simulink library "Lib_AC_AttitudeControl"  (R2014b)
settings: Solver=ode45  StartTime=0.0  StopTime=10.0  RelTol=1e-3
values from neighbouring files (symbols this model uses):
  Cutoff_frequency_roll = 20.0    (= 20)    [LoadParameters.m]    (also in euler_yaw_rate_cd.mat)
  Cutoff_frequency_yaw = 20.0    (= 20)    [LoadParameters.m]
  Discretetime_400Hz = 0.0025    [LoadParameters.m]    (also in euler_yaw_rate_cd.mat)
  roll_rate_kd = 0.0027    [LoadParameters.m]    (also in euler_yaw_rate_cd.mat = 0)
  roll_rate_ki = 0.001    [LoadParameters.m]    (also in euler_yaw_rate_cd.mat = 0)
  roll_rate_kp = 0.12    [LoadParameters.m]    (also in euler_yaw_rate_cd.mat = 0.08)
  yaw_rate_kd = 0.0090    (= 0.009)    [LoadParameters.m]
  yaw_rate_ki = 1.050    (= 1.05)    [LoadParameters.m]
  yaw_rate_kp = 0.45    [LoadParameters.m]
libraries: Lib_AC_PID x3
settings Model: Creator=Ehang  LastModifiedBy=Ehang

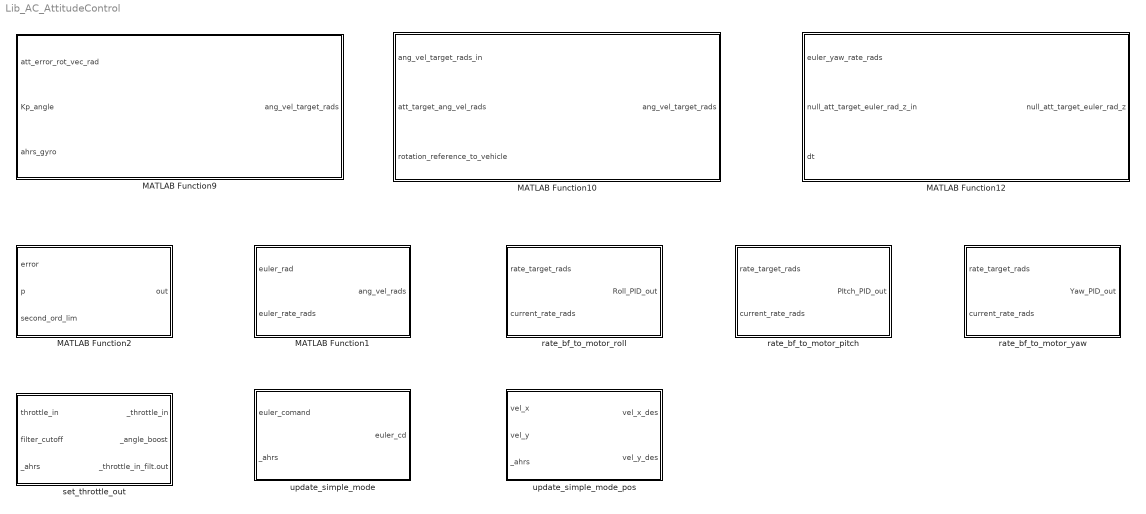
== system Lib_AC_AttitudeControl ==
  MATLAB Function1 : MATLAB Function  TreatAsAtomicUnit=on
  MATLAB Function10 : MATLAB Function  TreatAsAtomicUnit=on
  MATLAB Function12 : MATLAB Function  TreatAsAtomicUnit=on
  MATLAB Function2 : MATLAB Function  TreatAsAtomicUnit=on
  MATLAB Function9 : MATLAB Function  TreatAsAtomicUnit=on
  rate_bf_to_motor_pitch : Subsystem
  rate_bf_to_motor_roll : Subsystem
  rate_bf_to_motor_yaw : Subsystem
  set_throttle_out : Subsystem
  update_simple_mode : Subsystem
  update_simple_mode_pos : Subsystem

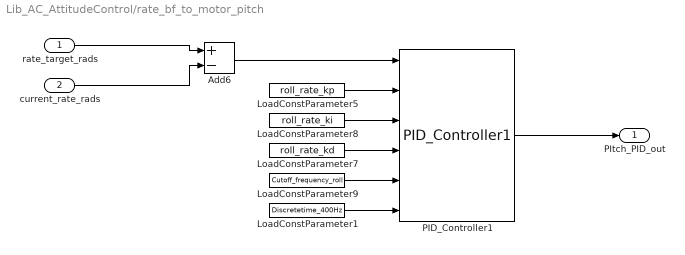
== system Lib_AC_AttitudeControl/rate_bf_to_motor_pitch ==
  rate_target_rads : Inport
  current_rate_rads : Inport  Port=2
  Add6 : Sum  Inputs=+-
  LoadConstParameter1 : Constant  Value=Discretetime_400Hz  SampleTime=-1
  LoadConstParameter5 : Constant  Value=roll_rate_kp  SampleTime=-1
  LoadConstParameter7 : Constant  Value=roll_rate_kd  SampleTime=-1
  LoadConstParameter8 : Constant  Value=roll_rate_ki  SampleTime=-1
  LoadConstParameter9 : Constant  Value=Cutoff_frequency_roll  SampleTime=-1
  PID_Controller1 : Lib_AC_PID/PID_Controller1  Description=PI控制器。
  PItch_PID_out : Outport
  wires:
  PID_Controller1/1 -> PItch_PID_out/1
  LoadConstParameter1/1 -> PID_Controller1/6
  LoadConstParameter9/1 -> PID_Controller1/5
  LoadConstParameter7/1 -> PID_Controller1/4
  LoadConstParameter8/1 -> PID_Controller1/3
  LoadConstParameter5/1 -> PID_Controller1/2
  Add6/1 -> PID_Controller1/1
  current_rate_rads/1 -> Add6/2
  rate_target_rads/1 -> Add6/1

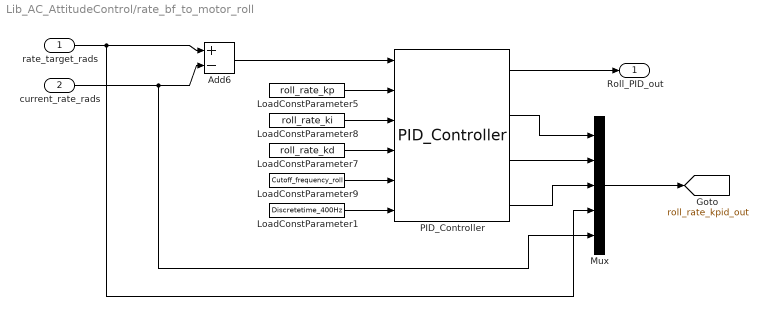
== system Lib_AC_AttitudeControl/rate_bf_to_motor_roll ==
  rate_target_rads : Inport
  current_rate_rads : Inport  Port=2
  Add6 : Sum  Inputs=+-
  LoadConstParameter1 : Constant  Value=Discretetime_400Hz  SampleTime=-1
  LoadConstParameter5 : Constant  Value=roll_rate_kp  SampleTime=-1
  LoadConstParameter7 : Constant  Value=roll_rate_kd  SampleTime=-1
  LoadConstParameter8 : Constant  Value=roll_rate_ki  SampleTime=-1
  LoadConstParameter9 : Constant  Value=Cutoff_frequency_roll  SampleTime=-1
  Mux : Mux  Inputs=5
  PID_Controller : Lib_AC_PID/PID_Controller  Description=PI控制器。
  Roll_PID_out : Outport
  tag scope: roll_rate_kpid_out=global
  wires:
  Mux/1 -> [roll_rate_kpid_out]
  PID_Controller/4 -> Mux/3
  PID_Controller/2 -> Mux/1
  PID_Controller/3 -> Mux/2
  PID_Controller/1 -> Roll_PID_out/1
  LoadConstParameter1/1 -> PID_Controller/6
  LoadConstParameter9/1 -> PID_Controller/5
  LoadConstParameter7/1 -> PID_Controller/4
  LoadConstParameter8/1 -> PID_Controller/3
  LoadConstParameter5/1 -> PID_Controller/2
  Add6/1 -> PID_Controller/1
  current_rate_rads/1 -> Mux/5, Add6/2
  rate_target_rads/1 -> Mux/4, Add6/1

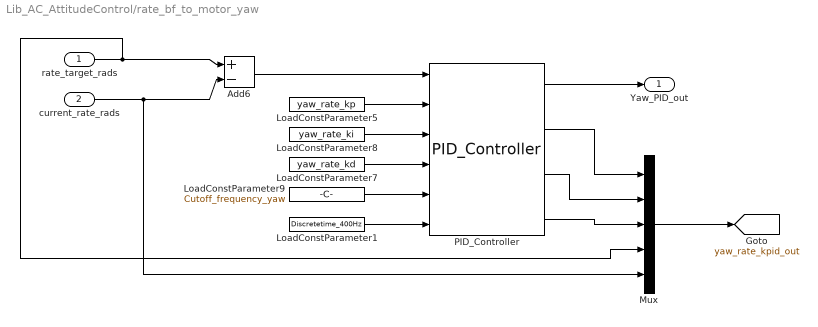
== system Lib_AC_AttitudeControl/rate_bf_to_motor_yaw ==
  rate_target_rads : Inport
  current_rate_rads : Inport  Port=2
  Add6 : Sum  Inputs=+-
  LoadConstParameter1 : Constant  Value=Discretetime_400Hz  SampleTime=-1
  LoadConstParameter5 : Constant  Value=yaw_rate_kp  SampleTime=-1
  LoadConstParameter7 : Constant  Value=yaw_rate_kd  SampleTime=-1
  LoadConstParameter8 : Constant  Value=yaw_rate_ki  SampleTime=-1
  LoadConstParameter9 : Constant  Value=Cutoff_frequency_yaw  SampleTime=-1
  Mux : Mux  Inputs=5
  PID_Controller : Lib_AC_PID/PID_Controller  Description=PI控制器。
  Yaw_PID_out : Outport
  tag scope: yaw_rate_kpid_out=global
  wires:
  PID_Controller/1 -> Yaw_PID_out/1
  LoadConstParameter1/1 -> PID_Controller/6
  LoadConstParameter9/1 -> PID_Controller/5
  LoadConstParameter7/1 -> PID_Controller/4
  LoadConstParameter8/1 -> PID_Controller/3
  LoadConstParameter5/1 -> PID_Controller/2
  Add6/1 -> PID_Controller/1
  current_rate_rads/1 -> Mux/5, Add6/2
  rate_target_rads/1 -> Mux/4, Add6/1
  Mux/1 -> [yaw_rate_kpid_out]
  PID_Controller/2 -> Mux/1
  PID_Controller/3 -> Mux/2
  PID_Controller/4 -> Mux/3

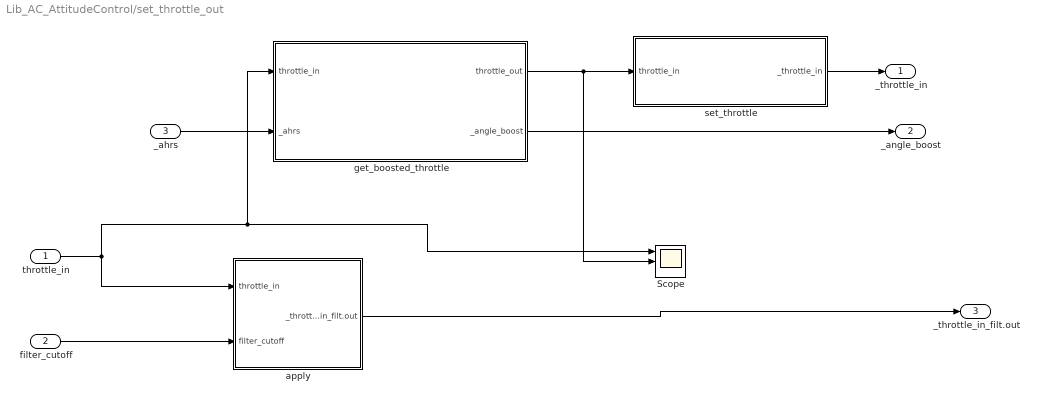
== system Lib_AC_AttitudeControl/set_throttle_out ==
  throttle_in : Inport
  filter_cutoff : Inport  Port=2
  _ahrs : Inport  Port=3
  Scope : Scope  NumInputPorts=3
      settings: YMin=-5~-5~-5  YMax=5~5~5  SaveName=ScopeData17
  apply : Subsystem
  get_boosted_throttle : Subsystem
  set_throttle : Subsystem
  _throttle_in : Outport
  _angle_boost : Outport  Port=2
  _throttle_in_filt.out : Outport  Port=3
  wires:
  _ahrs/1 -> get_boosted_throttle/2(_ahrs)
  get_boosted_throttle/1(throttle_out) -> Scope/2, set_throttle/1(throttle_in)
  set_throttle/1(_throttle_in) -> _throttle_in/1
  throttle_in/1 -> get_boosted_throttle/1(throttle_in), Scope/1, apply/1(throttle_in)
  filter_cutoff/1 -> apply/2(filter_cutoff)
  apply/1(_throttle_in_filt.out) -> _throttle_in_filt.out/1
  get_boosted_throttle/2(_angle_boost) -> _angle_boost/1

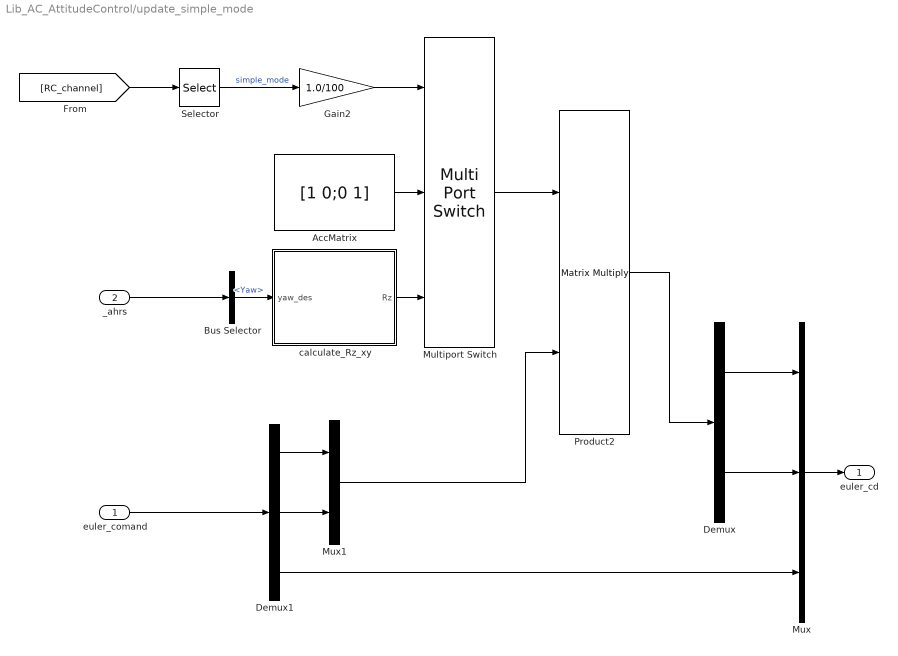
== system Lib_AC_AttitudeControl/update_simple_mode ==
  euler_comand : Inport
  _ahrs : Inport  Port=2
  AccMatrix : Constant  Value=[1 0;0 1]
  Bus Selector : BusSelector  OutputSignals=NEDState.Attitude.Yaw
  Demux : Demux  Outputs=2
  Demux1 : Demux  Outputs=3
  Gain2 : Gain  Gain=1.0/100
  Multiport Switch : MultiPortSwitch  Inputs=2
  Mux : Mux  Inputs=3
  Mux1 : Mux  Inputs=2
  Product2 : Product  Multiplication=Matrix(*)
  Selector : Selector  InputPortWidth=6  Indices=[6]
  calculate_Rz_xy : MATLAB Function  TreatAsAtomicUnit=on
  euler_cd : Outport
  wires:
  [RC_channel] -> Selector/1
  Selector/1 -> Gain2/1  "simple_mode"
  _ahrs/1 -> Bus Selector/1
  Bus Selector/1 -> calculate_Rz_xy/1(yaw_des)  "<Yaw>"
  calculate_Rz_xy/1(Rz) -> Multiport Switch/3
  AccMatrix/1 -> Multiport Switch/2
  Multiport Switch/1 -> Product2/1
  Product2/1 -> Demux/1
  Mux1/1 -> Product2/2
  euler_comand/1 -> Demux1/1
  Mux/1 -> euler_cd/1
  Demux1/3 -> Mux/3
  Demux1/1 -> Mux1/1
  Demux1/2 -> Mux1/2
  Demux/1 -> Mux/1
  Demux/2 -> Mux/2
  Gain2/1 -> Multiport Switch/1

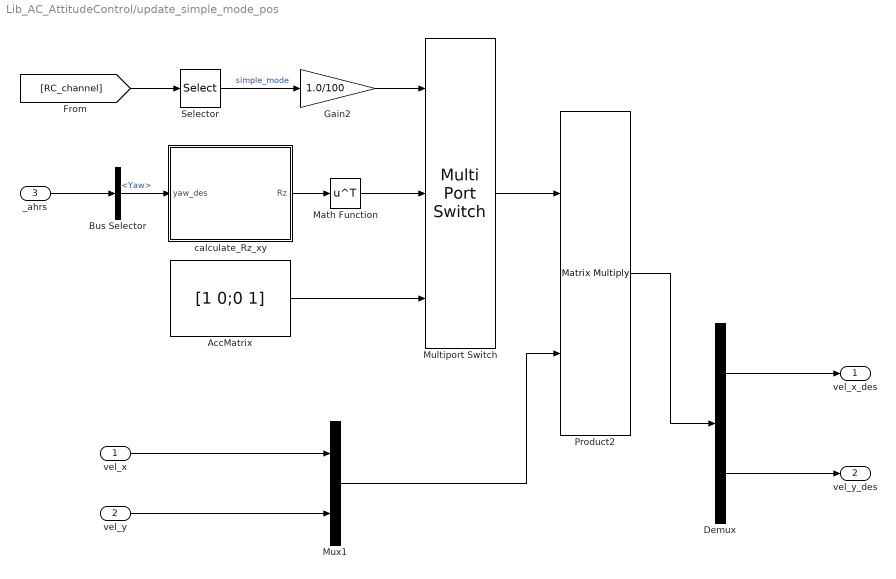
== system Lib_AC_AttitudeControl/update_simple_mode_pos ==
  vel_x : Inport
  vel_y : Inport  Port=2
  _ahrs : Inport  Port=3
  AccMatrix : Constant  Value=[1 0;0 1]
  Bus Selector : BusSelector  OutputSignals=NEDState.Attitude.Yaw
  Demux : Demux  Outputs=2
  Gain2 : Gain  Gain=1.0/100
  Math Function : Math  Operator=transpose  SaturateOnIntegerOverflow=on
  Multiport Switch : MultiPortSwitch  Inputs=2
  Mux1 : Mux  Inputs=2
  Product2 : Product  Multiplication=Matrix(*)
  Selector : Selector  InputPortWidth=6  Indices=[6]
  calculate_Rz_xy : MATLAB Function  TreatAsAtomicUnit=on
  vel_x_des : Outport
  vel_y_des : Outport  Port=2
  wires:
  Gain2/1 -> Multiport Switch/1
  Demux/2 -> vel_y_des/1
  vel_y/1 -> Mux1/2
  vel_x/1 -> Mux1/1
  Demux/1 -> vel_x_des/1
  Mux1/1 -> Product2/2
  Product2/1 -> Demux/1
  Multiport Switch/1 -> Product2/1
  calculate_Rz_xy/1(Rz) -> Math Function/1
  Bus Selector/1 -> calculate_Rz_xy/1(yaw_des)  "<Yaw>"
  _ahrs/1 -> Bus Selector/1
  Selector/1 -> Gain2/1  "simple_mode"
  [RC_channel] -> Selector/1
  Math Function/1 -> Multiport Switch/2
  AccMatrix/1 -> Multiport Switch/3

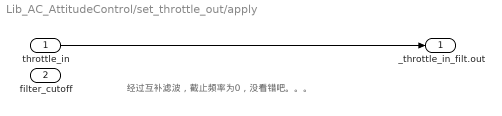
== system Lib_AC_AttitudeControl/set_throttle_out/apply ==
  note: 经过互补滤波，截止频率为0，没看错吧。。。
  throttle_in : Inport
  filter_cutoff : Inport  Port=2
  _throttle_in_filt.out : Outport
  wires:
  throttle_in/1 -> _throttle_in_filt.out/1

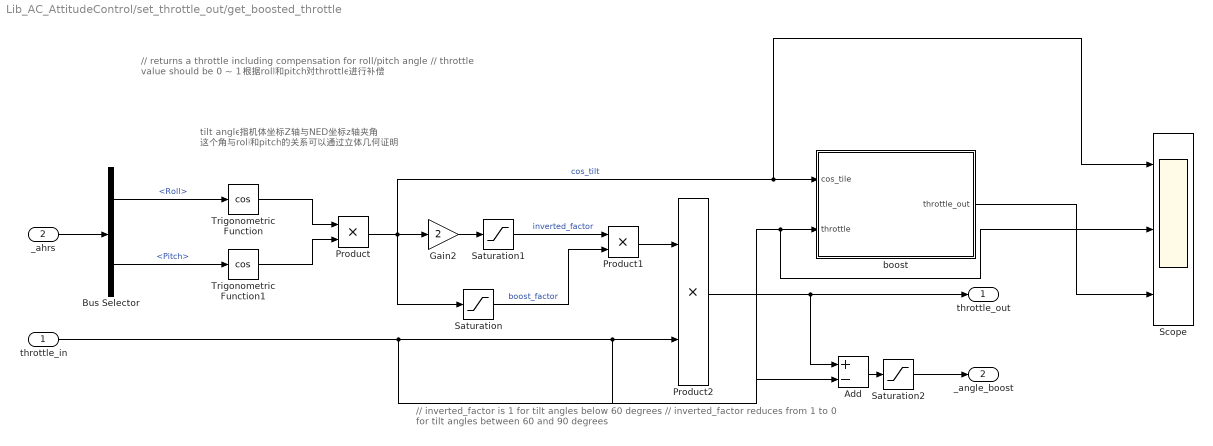
== system Lib_AC_AttitudeControl/set_throttle_out/get_boosted_throttle ==
  note: // inverted_factor is 1 for tilt angles below 60 degrees
      |     // inverted_factor reduces from 1 to 0 for tilt angles between 60 and 90 degrees
  note: tilt angle指机体坐标Z轴与NED坐标z轴夹角
      | 这个角与roll和pitch的关系可以通过立体几何证明
  note: // returns a throttle including compensation for roll/pitch angle
      | // throttle value should be 0 ~ 1 根据roll和pitch对throttle进行补偿
  throttle_in : Inport
  _ahrs : Inport  Port=2
  Add : Sum  Inputs=+-
  Bus Selector : BusSelector  OutputSignals=NEDState.Attitude.Roll,NEDState.Attitude.Pitch
  Gain2 : Gain  Gain=2
  Product : Product
  Product1 : Product
  Product2 : Product
  Saturation : Saturate  UpperLimit=1  LowerLimit=0.5
  Saturation1 : Saturate  UpperLimit=1  LowerLimit=0
  Saturation2 : Saturate  UpperLimit=1  LowerLimit=-1
  Scope : Scope  NumInputPorts=3
      settings: YMin=-5~-5~-5  YMax=5~5~5  SaveName=ScopeData6
  Trigonometric Function : Trigonometry  Operator=cos
  Trigonometric Function1 : Trigonometry  Operator=cos
  boost : Stateflow chart  TreatAsAtomicUnit=on
  throttle_out : Outport
  _angle_boost : Outport  Port=2
  wires:
  _ahrs/1 -> Bus Selector/1
  Bus Selector/1 -> Trigonometric Function/1  "<Roll>"
  Bus Selector/2 -> Trigonometric Function1/1  "<Pitch>"
  Trigonometric Function/1 -> Product/1
  Trigonometric Function1/1 -> Product/2
  Product/1 -> Scope/1, boost/1(cos_tile), Saturation/1, Gain2/1  "cos_tilt"
  throttle_in/1 -> Scope/2, boost/2(throttle), Add/2, Product2/2
  Gain2/1 -> Saturation1/1
  Saturation1/1 -> Product1/1  "inverted_factor"
  Saturation/1 -> Product1/2  "boost_factor"
  Product1/1 -> Product2/1
  Product2/1 -> Add/1, throttle_out/1
  Add/1 -> Saturation2/1
  Saturation2/1 -> _angle_boost/1
  boost/1(throttle_out) -> Scope/3

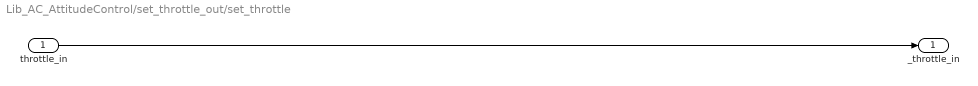
== system Lib_AC_AttitudeControl/set_throttle_out/set_throttle ==
  throttle_in : Inport
  _throttle_in : Outport
  wires:
  throttle_in/1 -> _throttle_in/1

== matlab function Lib_AC_AttitudeControl/MATLAB Function9 ==
  data: att_error_rot_vec_rad input; Kp_angle input; ang_vel_target_rads output; ahrs_gyro input size=[3,1]
function ang_vel_target_rads=update_ang_vel_target_from_att_error(att_error_rot_vec_rad,Kp_angle,ahrs_gyro)
%% 作用：根据大地坐标系下的旋转矢量误差，通过P控制器等输出机体坐标系下速度的期望。

%忽略判断语句
% p_angle_roll=25.5;
% p_angle_pitch=20.5;
% p_angle_yaw=10.5;
p_angle_roll=Kp_angle(1);
p_angle_pitch=Kp_angle(2);
p_angle_yaw=Kp_angle(3);
t_ang_vel_target_rads1 = p_angle_roll* att_error_rot_vec_rad(1);
t_ang_vel_target_rads2 = p_angle_pitch* att_error_rot_vec_rad(2);
t_ang_vel_target_rads3 = p_angle_yaw* att_error_rot_vec_rad(3);
 %     // Add feedforward term that attempts to ensure that the copter yaws about the reference
%     // Z axis, rather than the vehicle body Z axis.
%     // NOTE: This is a small-angle approximation.小角度近视，详细推到见caculate1
  t_ang_vel_target_rads1 =t_ang_vel_target_rads1 +att_error_rot_vec_rad(2) *ahrs_gyro(3);
  t_ang_vel_target_rads2 =t_ang_vel_target_rads2 -att_error_rot_vec_rad(1) *ahrs_gyro(3);
  
ang_vel_target_rads=[t_ang_vel_target_rads1,t_ang_vel_target_rads2,t_ang_vel_target_rads3]';

% void AC_AttitudeControl::update_ang_vel_target_from_att_error()
% {
%     // Compute the roll angular velocity demand from the roll angle error
%     if (_att_ctrl_use_accel_limit && _accel_roll_max > 0.0f) {
%         _ang_vel_target_rads.x = sqrt_controller(_att_error_rot_vec_rad.x, _p_angle_roll.kP(), constrain_float(get_accel_roll_max_radss()/2.0f,  AC_ATTITUDE_ACCEL_RP_CONTROLLER_MIN_RADSS, AC_ATTITUDE_ACCEL_RP_CONTROLLER_MAX_RADSS));
%     }else{//P控制
%     	//_att_error_rot_vec_rad 个人推到，这个参数与角速度期望成正比
%         _ang_vel_target_rads.x = _p_angle_roll.kP() * _att_error_rot_vec_rad.x;
%     }
% 
%     // Compute the pitch angular velocity demand from the roll angle error
%     if (_att_ctrl_use_accel_limit && _accel_pitch_max > 0.0f) {
%         _ang_vel_target_rads.y = sqrt_controller(_att_error_rot_vec_rad.y, _p_angle_pitch.kP(), constrain_float(get_accel_pitch_max_radss()/2.0f,  AC_ATTITUDE_ACCEL_RP_CONTROLLER_MIN_RADSS, AC_ATTITUDE_ACCEL_RP_CONTROLLER_MAX_RADSS));
%     }else{//P控制
%         _ang_vel_target_rads.y = _p_angle_pitch.kP() * _att_error_rot_vec_rad.y;
%     }
% 
%     // Compute the yaw angular velocity demand from the roll angle error
%     if (_att_ctrl_use_accel_limit && _accel_yaw_max > 0.0f) {
%         _ang_vel_target_rads.z = sqrt_controller(_att_error_rot_vec_rad.z, _p_angle_yaw.kP(), constrain_float(get_accel_yaw_max_radss()/2.0f,  AC_ATTITUDE_ACCEL_Y_CONTROLLER_MIN_RADSS, AC_ATTITUDE_ACCEL_Y_CONTROLLER_MAX_RADSS));
%     }else{
%         _ang_vel_target_rads.z = _p_angle_yaw.kP() * _att_error_rot_vec_rad.z;
%     }
% 
%     // Add feedforward term that attempts to ensure that the copter yaws about the reference
%     // Z axis, rather than the vehicle body Z axis.
%     // NOTE: This is a small-angle approximation.小角度近视？
%     //期望速率，通过角度误差校正？这是为什么？
%     _ang_vel_target_rads.x += _att_error_rot_vec_rad.y * _ahrs.get_gyro().z;
%     _ang_vel_target_rads.y += -_att_error_rot_vec_rad.x * _ahrs.get_gyro().z;
% }

== matlab function Lib_AC_AttitudeControl/MATLAB Function1 ==
  data: euler_rad input; euler_rate_rads input; ang_vel_rads output
function ang_vel_rads= euler_rate_to_ang_vel(euler_rad,euler_rate_rads)
%#codegen
% % 作用：将欧拉角的导数转化为B系下飞行器绕自身旋转的角速度。
%
     sin_theta = sin(euler_rad(2));
     cos_theta =cos(euler_rad(2));
     sin_phi = sin(euler_rad(1));
     cos_phi = cos(euler_rad(1));
    ang_vel_rads1 = euler_rate_rads(1) - sin_theta * euler_rate_rads(3);
    ang_vel_rads2 = cos_phi  * euler_rate_rads(2) + sin_phi * cos_theta * euler_rate_rads(3);
    ang_vel_rads3 = -sin_phi * euler_rate_rads(2) + cos_theta * cos_phi * euler_rate_rads(3);
    ang_vel_rads=[ang_vel_rads1;ang_vel_rads2;ang_vel_rads3];
%% 公式推到
% clear
% clc
% % cr:cos(roll)  sr:sin(roll)
% % cp:cos(pitch) sp:sin(pitch)
% % cy:cos(yaw)   sy:sin(yaw)
% syms cr sr cp sp cy sy
% % RZ:Rotate Z axis
% % RY:Rotate Y axis
% % RX:Rotate X axis
% syms  RZ RY RX
% %from earth to body
% % RZ:Rotate Z axis
% %右旋角度y为正
% RZ = [  cy   sy   0;
%        -sy   cy   0;
%         0    0    1];
% 
% % RY:Rotate Y axis
% %上仰角度P为正
% RY = [  cp   0  -sp;
%         0    1    0;
%         sp   0   cp];
% 
% % RX:Rotate X axis
% %右倾角度r为正
% RX = [  1    0    0;
%         0    cr  sr;
%         0   -sr  cr];
% %-----------------from_euler-----------------
% % column : a b c
% % row    : x y z
% %                    a                 b      c
% % x [            cp*cy,            cp*sy,   -sp]
% % y [ cy*sp*sr - cr*sy, cr*cy + sp*sr*sy, cp*sr]
% % z [ sr*sy + cr*cy*sp, cr*sp*sy - cy*sr, cp*cr]
% disp('Rotate Matix from earth fixed frame to body fixed frame;');
% from_euler = RX*RY*RZ
% %  yd  y的导数，pd  p的导数， rd r的导数
% %  [p,q,r]'表示B系下飞行器绕自身旋转的角速度。
% syms yd pd rd r p q
%  %rate_from_euler*[yd,pd,rd]'=[p,q,r]'
% rate_from_euler=RX*RY*[0;0;yd]+RX*[0;pd;0]+[rd;0;0];
% %        rd - sp*yd
% %  cr*pd + cp*sr*yd
% %  cp*cr*yd - pd*sr
% % [-sp,0,1][yd]
% % [cp*sr,cr,0][pd]
% % [cp*cr,-sr,0][rd]
% ab = [-sp      ,      0,      1;
%      cp*sr     ,     cr,      0;
%      cp*cr     ,    -sr,      0];
%  %[yd,pd,rd]'=from_rate*[p,q,r]'
%  disp('angle convert matix:');

% % 以下是Ｃ代码中的算法
% void AC_AttitudeControl::euler_rate_to_ang_vel(const Vector3f& euler_rad, const Vector3f& euler_rate_rads, Vector3f& ang_vel_rads)
% {
%      sin_theta = sinf(euler_rad.y);
%      cos_theta = cosf(euler_rad.y);
%      sin_phi = sinf(euler_rad.x);
%      cos_phi = cosf(euler_rad.x);
% 
%     ang_vel_rads.x = euler_rate_rads.x - sin_theta * euler_rate_rads.z;
%     ang_vel_rads.y = cos_phi  * euler_rate_rads.y + sin_phi * cos_theta * euler_rate_rads.z;
%     ang_vel_rads.z = -sin_phi * euler_rate_rads.y + cos_theta * cos_phi * euler_rate_rads.z;
% }

== matlab function Lib_AC_AttitudeControl/MATLAB Function2 ==
  data: error input; p input; out output; second_ord_lim input

function out=sqrt_controller(error,p,second_ord_lim)
linear_dist = second_ord_lim/(p*p);
    if error > linear_dist
        out=sqrt(2.0*second_ord_lim*(error-(linear_dist/2.0)));
    elseif error < -linear_dist 
        out=-sqrt(2.0*second_ord_lim*(-error-(linear_dist/2.0)));
    else 
        out=error*p;
    end

== matlab function Lib_AC_AttitudeControl/MATLAB Function10 ==
  data: ang_vel_target_rads_in input size=[3,1]; att_target_ang_vel_rads input size=[3,1]; ang_vel_target_rads output size=[3,1]; rotation_reference_to_vehicle input size=[3,3]

function ang_vel_target_rads=add_angular_velocity_feedforward(ang_vel_target_rads_in,att_target_ang_vel_rads,rotation_reference_to_vehicle)
%% 加入速率控制的前馈（前馈是以机体坐标系为参考）
% ang_vel_target_rads1=ang_vel_target_rads_in(1)+att_target_ang_vel_rads(1);
% ang_vel_target_rads2=ang_vel_target_rads_in(2)+att_target_ang_vel_rads(2);
% ang_vel_target_rads3=ang_vel_target_rads_in(3)+att_target_ang_vel_rads(3);
% ang_vel_target_rads=[ang_vel_target_rads1,ang_vel_target_rads2,ang_vel_target_rads3]';

ang_vel_target_rads=ang_vel_target_rads_in+rotation_reference_to_vehicle*att_target_ang_vel_rads;

% // Add the angular velocity feedforward, rotated into vehicle frame
%     Matrix3f Trv;
%     get_rotation_reference_to_vehicle(Trv);
%     _ang_vel_target_rads += Trv * _att_target_ang_vel_rads;

== stateflow chart Lib_AC_AttitudeControl/set_throttle_out/get_boosted_throttle/boost ==
  settings: updateMethod=DISCRETE  sampleTime=0.0025  initializeOutput=1
  note: %状态不变，输入数据就不更新，这个不解决，这个模块就无法用。。。
  state big_tile
    entry:
    throttle_out=4.0*cos_tile*throttle;
  state small_tile
    entry:
    throttle_out=throttle*1.0/cos_tile;
  big_tile -> small_tile : [cos_tile>0.9]
  (default) -> small_tile
  small_tile -> big_tile : [cos_tile<0.9]
  data: cos_tile input; throttle_out output double; throttle input double
  data cos_tile settings: description=飞机倾斜角余弦

== matlab function Lib_AC_AttitudeControl/update_simple_mode/calculate_Rz_xy ==
  data: Rz output size=[2,2]; yaw_des input
function Rz  = Rz_xy(yaw_des)
%#codegen
Rz=[ cos(yaw_des)  sin(yaw_des);
    -sin(yaw_des)  cos(yaw_des)];

== matlab function Lib_AC_AttitudeControl/update_simple_mode_pos/calculate_Rz_xy ==
  data: Rz output size=[2,2]; yaw_des input
function Rz  = Rz_xy(yaw_des)
%#codegen
Rz=[ cos(yaw_des)  sin(yaw_des);
    -sin(yaw_des)  cos(yaw_des)];

== matlab function Lib_AC_AttitudeControl/MATLAB Function12 ==
  data: euler_yaw_rate_rads input; null_att_target_euler_rad_z_in input; null_att_target_euler_rad_z output; dt input

function null_att_target_euler_rad_z=update_att_target_yaw(euler_yaw_rate_rads,null_att_target_euler_rad_z_in,dt)
null_att_target_euler_rad_z=null_att_target_euler_rad_z_in+euler_yaw_rate_rads * dt;
